simulink library "massignmentLib"  (Simulink 6.0)
settings: Solver=ode45  StartTime=0.0  StopTime=10.0  RelTol=1e-3
settings Model: Creator=awarlock  LastModifiedBy=awarlock  ExtModeAutoUpdateStatusClock=off
settings DebuggingCC: MultiTaskDSMMsg=warning

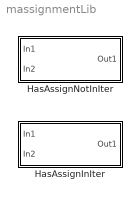
== system massignmentLib ==
  HasAssignInIter : Subsystem  TreatAsAtomicUnit=on
  HasAssignNotInIter : Subsystem  TreatAsAtomicUnit=on

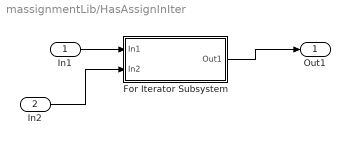
== system massignmentLib/HasAssignInIter ==
  In1 : Inport  Port=1  LatchInput=off
  In2 : Inport  Port=2  LatchInput=off
  For Iterator Subsystem : Subsystem  TreatAsAtomicUnit=on
  Out1 : Outport
  wires:
  In1/1 -> For Iterator Subsystem/1(In1)
  In2/1 -> For Iterator Subsystem/2(In2)
  For Iterator Subsystem/1(Out1) -> Out1/1

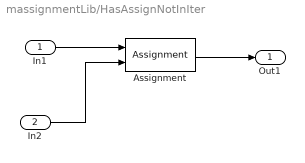
== system massignmentLib/HasAssignNotInIter ==
  In1 : Inport  Port=1  LatchInput=off
  In2 : Inport  Port=2  LatchInput=off
  Assignment : Assignment
  Out1 : Outport
  wires:
  In1/1 -> Assignment/1
  In2/1 -> Assignment/2
  Assignment/1 -> Out1/1

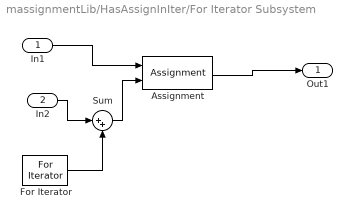
== system massignmentLib/HasAssignInIter/For Iterator Subsystem ==
  In1 : Inport  Port=1  LatchInput=off
  In2 : Inport  Port=2  LatchInput=off
  Assignment : Assignment
  For Iterator : ForIterator  IterationVariableDataType=double
  Sum : Sum  Inputs=|++
  Out1 : Outport
  wires:
  In2/1 -> Sum/1
  For Iterator/1 -> Sum/2
  In1/1 -> Assignment/1
  Sum/1 -> Assignment/2
  Assignment/1 -> Out1/1
